simulink model "Experiment"  (R2015b)
settings: configuration reference "ControlConfig" (kept outside this file)
values from neighbouring files (symbols this model uses):
  Ts = 0.02    [ControlInit.m]
undefined symbols (not defined in the file or in its folder): j
libraries: powerlib x11, simulink x5, powerlib_meascontrol x1
settings Model: Creator=Emilio  LastModifiedBy=Emilio
settings ConfigSetRef: SourceLocation=Base Workspace

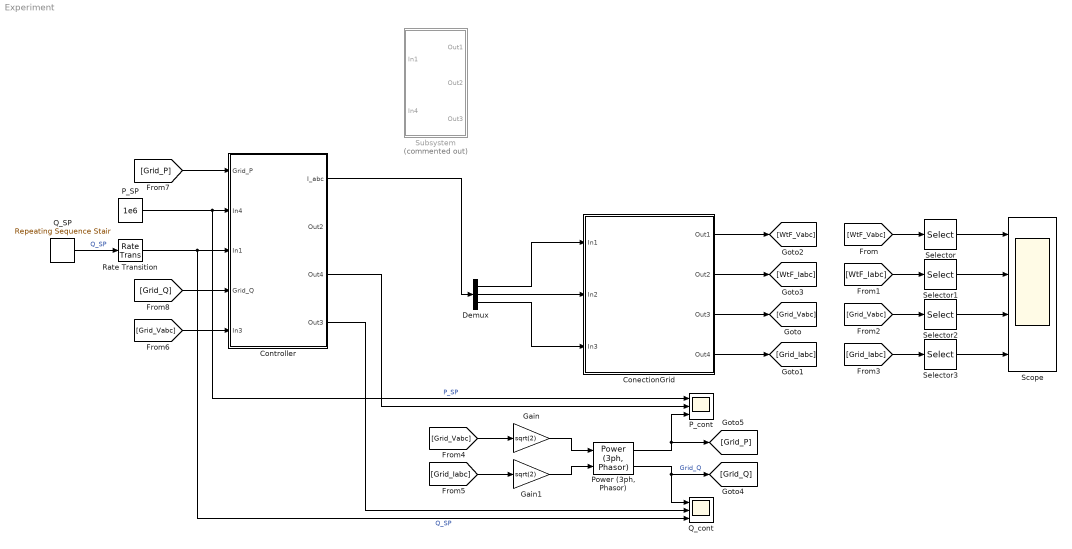
== system Experiment ==
  ConectionGrid : Subsystem
  Controller : Subsystem
  Demux : Demux  Outputs=3
  Gain : Gain  Gain=sqrt(2)
  Gain1 : Gain  Gain=sqrt(2)
  P_SP : Constant  Value=1e6
  P_cont : Scope  NumInputPorts=3
  "Power (3ph, Phasor)" : powerlib_meascontrol/Measurements/Power (3ph, Phasor)
  Q_SP : simulink/Sources/Repeating Sequence Stair  OutValues=[4e6 2e6 6e6 1e6].'  tsamp=5  OutMin=[]  OutMax=[]  OutDataTypeStr=double  OutputDataTypeScalingMode=double  OutDataType=fixdt(0,8)  ConRadixGroup=Best Precision: Vector-wise  OutScaling=2^-12
  Q_cont : Scope  NumInputPorts=3
  Rate Transition : RateTransition  OutPortSampleTime=Ts
  Scope : Scope  NumInputPorts=4
  Selector{,1..3} (4 alike) : Selector  InputPortWidth=3  IndexOptions=Index vector (dialog)  Indices=[1]  OutputSizes=1
  Subsystem : Subsystem  Commented=on
  wires:
  ConectionGrid/1(Out1) -> [WtF_Vabc]
  ConectionGrid/2(Out2) -> [WtF_Iabc]
  ConectionGrid/3(Out3) -> [Grid_Vabc]
  ConectionGrid/4(Out4) -> [Grid_Iabc]
  [WtF_Vabc] -> Selector/1
  [WtF_Iabc] -> Selector1/1
  [Grid_Vabc] -> Selector2/1
  [Grid_Iabc] -> Selector3/1
  Selector/1 -> Scope/1
  Selector1/1 -> Scope/2
  Selector2/1 -> Scope/3
  Selector3/1 -> Scope/4
  [Grid_Vabc] -> Gain/1
  [Grid_Iabc] -> Gain1/1
  Gain/1 -> "Power (3ph, Phasor)"/1
  Gain1/1 -> "Power (3ph, Phasor)"/2
  "Power (3ph, Phasor)"/1 -> [Grid_P], P_cont/3
  "Power (3ph, Phasor)"/2 -> Q_cont/1, [Grid_Q]  "Grid_Q"
  Q_SP/1 -> Rate Transition/1  "Q_SP"
  [Grid_Q] -> Controller/4(Grid_Q)
  [Grid_Vabc] -> Controller/5(In3)
  Controller/4(Out3) -> Q_cont/2
  P_SP/1 -> Controller/2(In4), P_cont/1  "P_SP"
  [Grid_P] -> Controller/1(Grid_P)
  Controller/3(Out4) -> P_cont/2
  Rate Transition/1 -> Q_cont/3, Controller/3(In1)  "Q_SP"
  Controller/1(I_abc) -> Demux/1
  Demux/1 -> ConectionGrid/1(In1)
  Demux/2 -> ConectionGrid/2(In2)
  Demux/3 -> ConectionGrid/3(In3)

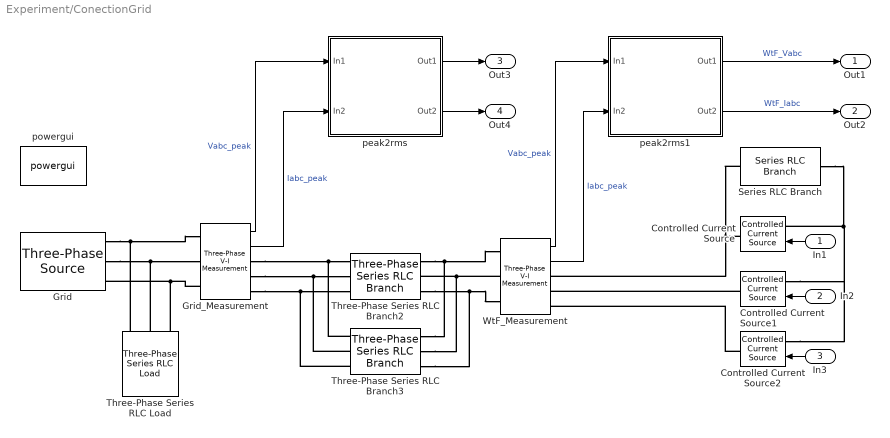
== system Experiment/ConectionGrid ==
  In1 : Inport
  In2 : Inport  Port=2
  In3 : Inport  Port=3
  Controlled Current Source : powerlib/Electrical Sources/Controlled Current Source  Initialize=on  Source_Type=AC  Amplitude=1  Phase=1  Frequency=50  Measurements=None
  Controlled Current Source1 : powerlib/Electrical Sources/Controlled Current Source  Initialize=on  Source_Type=AC  Amplitude=1  Phase=1  Frequency=50  Measurements=None
  Controlled Current Source2 : powerlib/Electrical Sources/Controlled Current Source  Initialize=on  Source_Type=AC  Amplitude=1  Phase=1  Frequency=50  Measurements=None
  Grid : powerlib/Electrical Sources/Three-Phase Source  InternalConnection=Yg  VoltagePhases=off  Voltage=400e3  PhaseAngle=0  Voltage_phases=[25e3 25e3 25e3]/sqrt(3)  PhaseAngles_phases=[0 -120 +120]  Frequency=50  NonIdealSource=on  SpecifyImpedance=on  Resistance=0.8929  Inductance=16.58e-3  ShortCircuitLevel=100e6  BaseVoltage=25e3  XRratio=7  BusType=swing  Pref=10e3  Qref=0  Prefabc=[10e3, 10e3, 10e3]  Qrefabc=[0, 0, 0]  Qmin=-inf  Qmax=inf
  Grid_Measurement : powerlib/Measurements/Three-Phase V-I Measurement  VoltageMeasurement=phase-to-ground  SetLabelV=off  LabelV=Vabc  Vpu=off  VpuLL=off  CurrentMeasurement=yes  SetLabelI=off  LabelI=Iabc  Ipu=off  Pbase=100e6  Vbase=500e3  OutputType=Complex  PhasorSimulation=on  PSBequivalent=0
  Series RLC Branch : powerlib/Elements/Series RLC Branch  LConnTagsString=__new0  RConnTagsString=__new0  BranchType=R  Resistance=10e10  Inductance=1e-3  SetiL0=off  InitialCurrent=0  Capacitance=1e-6  Setx0=off  InitialVoltage=0  Measurements=None
  Three-Phase Series RLC Branch2 : powerlib/Elements/Three-Phase Series RLC Branch  LConnTagsString=A|B|C  RConnTagsString=A|B|C  BranchType=RL  Resistance=10  Inductance=1e-5  Capacitance=0  Measurements=None
  Three-Phase Series RLC Branch3 : powerlib/Elements/Three-Phase Series RLC Branch  LConnTagsString=A|B|C  RConnTagsString=A|B|C  BranchType=R  Resistance=10e10  Inductance=1e-3  Capacitance=1e-6  Measurements=None
  Three-Phase Series RLC Load : powerlib/Elements/Three-Phase Series RLC Load  LConnTagsString=A|B|C  Configuration=Y (grounded)  NominalVoltage=1000  Vabc=[1e3 1e3 1e3]  Vabcp=[1e3 1e3 1e3]  NominalFrequency=60  UnbalancedPower=off  ActivePower=10  InductivePower=0  CapacitivePower=0  Pabc=[10e3 9e3 11e3]  QLabc=[100 90 110]  QCabc=[100 90 110]  Pabcp=[10e3 9e3 11e3]  QLabcp=[100 90 110]  QCabcp=[100 90 110]  Measurements=None  LoadType=constant Z
  WtF_Measurement : powerlib/Measurements/Three-Phase V-I Measurement  VoltageMeasurement=phase-to-ground  SetLabelV=off  LabelV=Vabc  Vpu=off  VpuLL=off  CurrentMeasurement=yes  SetLabelI=off  LabelI=Iabc  Ipu=off  Pbase=100e6  Vbase=500e3  OutputType=Complex  PhasorSimulation=on  PSBequivalent=0
  peak2rms : Subsystem
  peak2rms1 : Subsystem
  powergui : powerlib/powergui  Priority=1  SimulationMode=Phasor  SolverType=Tustin/Backward Euler (TBE)  SampleTime=50e-6  frequency=50  SPID=off  DisableSnubberDevices=off  DisableRonSwitches=off  DisableVfSwitches=off  SwTol=0  DisplayEquations=off  Interpol=off  ExternalGateDelay=off  methode=off  Ts=10  FunctionMessages=off  echomessages=off  HookPort=off  EnableUseOfTLC=off  x0status=blocks  frequencyindice=50  Pbase=100e6  ErrMax=1e-4  Iterations=50  UnitsV=kV  UnitsW=MW  buscounter=0  RestoreLinks=warning  ResistiveCurrentMeasurement=off  Frange=[0:2:500]  Ylog=off  Xlog=on  ShowGrid=off  save=off  variable=ZData  structure=0  ZoomFFT=off  StartTime=0.0  cycles=1  DisplayStyle=1  fundamental=60  FreqAxis=off  MaxFrequency=1000  frequencyindicesteady=1  RmsSteady=1  display=off
  Out1 : Outport
  Out2 : Outport  Port=2
  Out3 : Outport  Port=3
  Out4 : Outport  Port=4
  wires:
  peak2rms/1(Out1) -> Out3/1
  peak2rms/2(Out2) -> Out4/1
  Grid_Measurement/2 -> peak2rms/2(In2)  "Iabc_peak"
  Grid_Measurement/1 -> peak2rms/1(In1)  "Vabc_peak"
  WtF_Measurement/2 -> peak2rms1/2(In2)  "Iabc_peak"
  peak2rms1/1(Out1) -> Out1/1  "WtF_Vabc"
  peak2rms1/2(Out2) -> Out2/1  "WtF_Iabc"
  WtF_Measurement/1 -> peak2rms1/1(In1)  "Vabc_peak"
  In3/1 -> Controlled Current Source2/1
  In1/1 -> Controlled Current Source/1
  In2/1 -> Controlled Current Source1/1
  connections:
  Controlled Current Source1/RConn1 -- WtF_Measurement/RConn2
  Grid/RConn2 -- Three-Phase Series RLC Load/LConn2 -- Grid_Measurement/LConn2
  Grid_Measurement/RConn2 -- Three-Phase Series RLC Branch3/LConn2 -- Three-Phase Series RLC Branch2/LConn2
  Grid_Measurement/RConn3 -- Three-Phase Series RLC Branch3/LConn3 -- Three-Phase Series RLC Branch2/LConn3
  Controlled Current Source/RConn1 -- Series RLC Branch/LConn1 -- WtF_Measurement/RConn1
  WtF_Measurement/LConn2 -- Three-Phase Series RLC Branch3/RConn2 -- Three-Phase Series RLC Branch2/RConn2
  Controlled Current Source2/LConn1 -- Controlled Current Source1/LConn1 -- Series RLC Branch/RConn1 -- Controlled Current Source/LConn1
  Three-Phase Series RLC Branch2/RConn3 -- Three-Phase Series RLC Branch3/RConn3 -- WtF_Measurement/LConn3
  Controlled Current Source2/RConn1 -- WtF_Measurement/RConn3
  Three-Phase Series RLC Branch2/RConn1 -- WtF_Measurement/LConn1 -- Three-Phase Series RLC Branch3/RConn1
  Grid_Measurement/LConn3 -- Three-Phase Series RLC Load/LConn3 -- Grid/RConn3
  Grid_Measurement/RConn1 -- Three-Phase Series RLC Branch3/LConn1 -- Three-Phase Series RLC Branch2/LConn1
  Grid/RConn1 -- Three-Phase Series RLC Load/LConn1 -- Grid_Measurement/LConn1

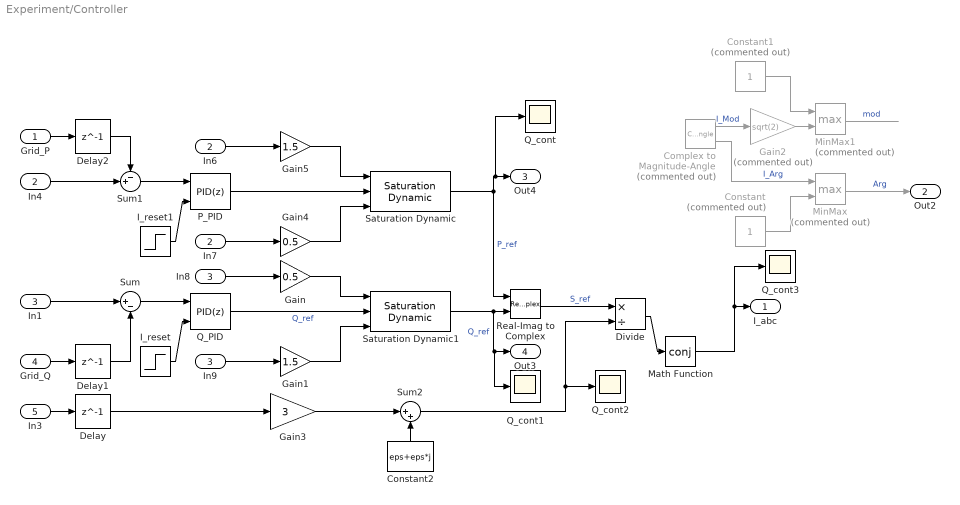
== system Experiment/Controller ==
  Grid_P : Inport
  In4 : Inport  Port=2
  In1 : Inport  Port=3
  Grid_Q : Inport  Port=4
  In3 : Inport  Port=5
  Complex to Magnitude-Angle : ComplexToMagnitudeAngle  Commented=on
  Constant : Constant  Commented=on
  Constant1 : Constant  Commented=on
  Constant2 : Constant  Value=eps+eps*j
  Delay : Delay  DelayLength=1  InitialCondition=0
  Delay1 : Delay  DelayLength=1  InitialCondition=0
  Delay2 : Delay  DelayLength=1  InitialCondition=0
  Divide : Product  Inputs=*/
  Gain : Gain  Gain=0.5
  Gain1 : Gain  Gain=1.5
  Gain2 : Gain  Commented=on  Gain=sqrt(2)
  Gain3 : Gain  Gain=3
  Gain4 : Gain  Gain=0.5
  Gain5 : Gain  Gain=1.5
  I_reset : Step  Time=5  SampleTime=Ts
  I_reset1 : Step  Time=5  SampleTime=Ts
  In6 : InportShadow  Port=2
  In7 : InportShadow  Port=2
  In8 : InportShadow  Port=3
  In9 : InportShadow  Port=3
  Math Function : Math  Operator=conj  SaturateOnIntegerOverflow=on
  MinMax : MinMax  Commented=on  Function=max  Inputs=2
  MinMax1 : MinMax  Commented=on  Function=max  Inputs=2
  P_PID : simulink/Continuous/PID Controller  Controller=PID  TimeDomain=Discrete-time  SampleTime=Ts  IntegratorMethod=Forward Euler  FilterMethod=Forward Euler  Form=Parallel  UseFilter=on  ControllerParametersSource=internal  P=0.25  I=7.5  D=0  N=100  InitialConditionSource=internal  InitialConditionForIntegrator=0  InitialConditionForFilter=0  ExternalReset=either  LimitOutput=off  UpperSaturationLimit=inf  LowerSaturationLimit=-inf  LinearizeAsGain=off  AntiWindupMode=none  Kb=1  TrackingMode=off  Kt=1  PParamMin=[]  PParamMax=[]  IParamMin=[]  IParamMax=[]  DParamMin=[]  DParamMax=[]  NParamMin=[]  NParamMax=[]  KbParamMin=[]  KbParamMax=[]  KtParamMin=[]  KtParamMax=[]  POutMin=[]  POutMax=[]  IOutMin=[]  IOutMax=[]  DOutMin=[]  DOutMax=[]  NOutMin=[]  NOutMax=[]  KbOutMin=[]  KbOutMax=[]  KtOutMin=[]  KtOutMax=[]  IntegratorOutMin=[]  IntegratorOutMax=[]  FilterOutMin=[]  FilterOutMax=[]  SumOutMin=[]  SumOutMax=[]  SumI1OutMin=[]  SumI1OutMax=[]  SumI2OutMin=[]  SumI2OutMax=[]  SumI3OutMin=[]  SumI3OutMax=[]  SumDOutMin=[]  SumDOutMax=[]  SaturationOutMin=[]  SaturationOutMax=[]  IntegratorContinuousStateAttributes=''  IntegratorStateMustResolveToSignalObject=off  IntegratorRTWStateStorageClass=Auto  FilterContinuousStateAttributes=''  FilterStateMustResolveToSignalObject=off  FilterRTWStateStorageClass=Auto  DifferentiatorICPrevScaledInput=0  DifferentiatorOutMin=[]  DifferentiatorOutMax=[]
  Q_PID : simulink/Continuous/PID Controller  Controller=PID  TimeDomain=Discrete-time  SampleTime=Ts  IntegratorMethod=Forward Euler  FilterMethod=Forward Euler  Form=Parallel  UseFilter=on  ControllerParametersSource=internal  P=0.5  I=2  D=0  N=100  InitialConditionSource=internal  InitialConditionForIntegrator=0  InitialConditionForFilter=0  ExternalReset=rising  LimitOutput=off  UpperSaturationLimit=inf  LowerSaturationLimit=-inf  LinearizeAsGain=off  AntiWindupMode=none  Kb=1  TrackingMode=off  Kt=1  PParamMin=[]  PParamMax=[]  IParamMin=[]  IParamMax=[]  DParamMin=[]  DParamMax=[]  NParamMin=[]  NParamMax=[]  KbParamMin=[]  KbParamMax=[]  KtParamMin=[]  KtParamMax=[]  POutMin=[]  POutMax=[]  IOutMin=[]  IOutMax=[]  DOutMin=[]  DOutMax=[]  NOutMin=[]  NOutMax=[]  KbOutMin=[]  KbOutMax=[]  KtOutMin=[]  KtOutMax=[]  IntegratorOutMin=[]  IntegratorOutMax=[]  FilterOutMin=[]  FilterOutMax=[]  SumOutMin=[]  SumOutMax=[]  SumI1OutMin=[]  SumI1OutMax=[]  SumI2OutMin=[]  SumI2OutMax=[]  SumI3OutMin=[]  SumI3OutMax=[]  SumDOutMin=[]  SumDOutMax=[]  SaturationOutMin=[]  SaturationOutMax=[]  IntegratorContinuousStateAttributes=''  IntegratorStateMustResolveToSignalObject=off  IntegratorRTWStateStorageClass=Auto  FilterContinuousStateAttributes=''  FilterStateMustResolveToSignalObject=off  FilterRTWStateStorageClass=Auto  DifferentiatorICPrevScaledInput=0  DifferentiatorOutMin=[]  DifferentiatorOutMax=[]
  Q_cont{,1..3} (4 alike) : Scope
  Real-Imag to Complex : RealImagToComplex
  Saturation Dynamic : simulink/Discontinuities/Saturation Dynamic  OutMin=[]  OutMax=[]  OutDataTypeStr=Inherit: Same as second input  OutDataType=fixdt(1, 16)  OutScaling=2^-10  DoSatur=off
  Saturation Dynamic1 : simulink/Discontinuities/Saturation Dynamic  OutMin=[]  OutMax=[]  OutDataTypeStr=Inherit: Same as second input  OutDataType=fixdt(1, 16)  OutScaling=2^-10  DoSatur=off
  Sum : Sum  Inputs=|+-
  Sum1 : Sum  Inputs=-+|
  Sum2 : Sum  Inputs=|++
  I_abc : Outport
  Out2 : Outport  Port=2
  Out4 : Outport  Port=3
  Out3 : Outport  Port=4
  wires:
  Real-Imag to Complex/1 -> Divide/1  "S_ref"
  Grid_Q/1 -> Delay1/1
  Delay/1 -> Gain3/1
  Complex to Magnitude-Angle/2 -> MinMax/1  "I_Arg"
  In3/1 -> Delay/1
  Complex to Magnitude-Angle/1 -> Gain2/1  "I_Mod"
  Sum/1 -> Q_PID/1
  MinMax1/1 -> ?  "mod"
  Divide/1 -> Math Function/1
  MinMax/1 -> Out2/1  "Arg"
  In1/1 -> Sum/1
  Delay1/1 -> Sum/2
  Constant/1 -> MinMax/2
  Gain2/1 -> MinMax1/2
  Constant1/1 -> MinMax1/1
  Math Function/1 -> Q_cont3/1, I_abc/1
  Saturation Dynamic1/1 -> Real-Imag to Complex/2, Q_cont1/1, Out3/1  "Q_ref"
  Saturation Dynamic/1 -> Real-Imag to Complex/1, Q_cont/1, Out4/1  "P_ref"
  Sum1/1 -> P_PID/1
  In4/1 -> Sum1/2
  Grid_P/1 -> Delay2/1
  Delay2/1 -> Sum1/1
  I_reset/1 -> Q_PID/2
  I_reset1/1 -> P_PID/2
  Gain3/1 -> Sum2/1
  Constant2/1 -> Sum2/2
  Sum2/1 -> Q_cont2/1, Divide/2
  P_PID/1 -> Saturation Dynamic/2
  Q_PID/1 -> Saturation Dynamic1/2  "Q_ref"
  In8/1 -> Gain/1
  Gain/1 -> Saturation Dynamic1/1
  In9/1 -> Gain1/1
  Gain1/1 -> Saturation Dynamic1/3
  In7/1 -> Gain4/1
  Gain4/1 -> Saturation Dynamic/3
  In6/1 -> Gain5/1
  Gain5/1 -> Saturation Dynamic/1

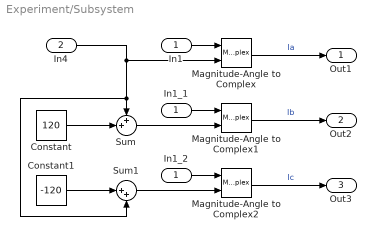
== system Experiment/Subsystem ==
  In1 : Inport
  In4 : Inport  Port=2
  Constant : Constant  Value=120
  Constant1 : Constant  Value=-120
  In1_1 : InportShadow
  In1_2 : InportShadow
  Magnitude-Angle to Complex : MagnitudeAngleToComplex
  Magnitude-Angle to Complex1 : MagnitudeAngleToComplex
  Magnitude-Angle to Complex2 : MagnitudeAngleToComplex
  Sum : Sum  Inputs=++|
  Sum1 : Sum  Inputs=|++
  Out1 : Outport
  Out2 : Outport  Port=2
  Out3 : Outport  Port=3
  wires:
  Constant/1 -> Sum/2
  Magnitude-Angle to Complex1/1 -> Out2/1  "Ib"
  In1_1/1 -> Magnitude-Angle to Complex1/1
  Magnitude-Angle to Complex2/1 -> Out3/1  "Ic"
  Magnitude-Angle to Complex/1 -> Out1/1  "Ia"
  In1/1 -> Magnitude-Angle to Complex/1
  Sum/1 -> Magnitude-Angle to Complex1/2
  In4/1 -> Magnitude-Angle to Complex/2, Sum1/2, Sum/1
  Constant1/1 -> Sum1/1
  Sum1/1 -> Magnitude-Angle to Complex2/2
  In1_2/1 -> Magnitude-Angle to Complex2/1

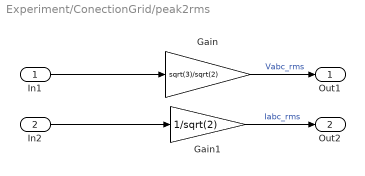
== system Experiment/ConectionGrid/peak2rms ==
  In1 : Inport
  In2 : Inport  Port=2
  Gain : Gain  Gain=sqrt(3)/sqrt(2)
  Gain1 : Gain  Gain=1/sqrt(2)
  Out1 : Outport
  Out2 : Outport  Port=2
  wires:
  Gain/1 -> Out1/1  "Vabc_rms"
  In1/1 -> Gain/1
  Gain1/1 -> Out2/1  "Iabc_rms"
  In2/1 -> Gain1/1

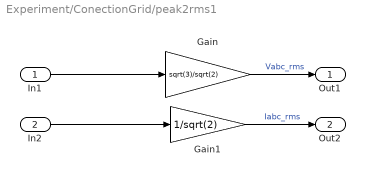
== system Experiment/ConectionGrid/peak2rms1 ==
  In1 : Inport
  In2 : Inport  Port=2
  Gain : Gain  Gain=sqrt(3)/sqrt(2)
  Gain1 : Gain  Gain=1/sqrt(2)
  Out1 : Outport
  Out2 : Outport  Port=2
  wires:
  In2/1 -> Gain1/1
  Gain1/1 -> Out2/1  "Iabc_rms"
  In1/1 -> Gain/1
  Gain/1 -> Out1/1  "Vabc_rms"
